simulink model "VVI"  (R2020a)
settings: Solver=FixedStepAuto  StartTime=0.0  StopTime=10.0  FixedStep=1e-3  RelTol=1e-3  EnableMultiTasking=on
undefined symbols (not defined in the file): D1, D10, D12, D13, D2, D3, D5, D7, D9, PTA1, PTA2, PTB9, PTC17, PTC3, PTC4, PTD0, PTD1, PTD3
libraries: frdmk64flib x11
settings Model: ExtModeTrigDuration=5  Creator=guga  LastModifiedBy=guga
settings OptimizationCC: EnhancedBackFolding=on  PassReuseOutputArgsAs=Individual arguments  ZeroExternalMemoryAtStartup=off  ZeroInternalMemoryAtStartup=off  MaxStackSize=64  OptimizeBlockOrder=speed  DifferentSizesBufferReuse=on  OptimizationCustomize=off  EfficientTunableParamExpr=on
settings DebuggingCC: ParameterTunabilityLossMsg=error
settings HardwareCC: ProdBitPerPointer=32  ProdBitPerSizeT=32  ProdBitPerPtrDiffT=32  ProdLargestAtomicInteger=Long  ProdLargestAtomicFloat=Double  ProdWordSize=32  ProdHWDeviceType=ARM Compatible->ARM Cortex
settings SFSimCC: MATLABDynamicMemAlloc=off
settings RTWCC: SystemTargetFile=ert.tlc  HardwareBoard=NXP FRDM-K64F  TemplateMakefile=ert_default_tmf  Toolchain=GNU Tools for ARM Embedded Processors
settings CodeAppCC: ForceParamTrailComments=on  IgnoreCustomStorageClasses=off  OperatorAnnotations=on  SimulinkDataObjDesc=on  SFDataObjDesc=on  InsertBlockDesc=on

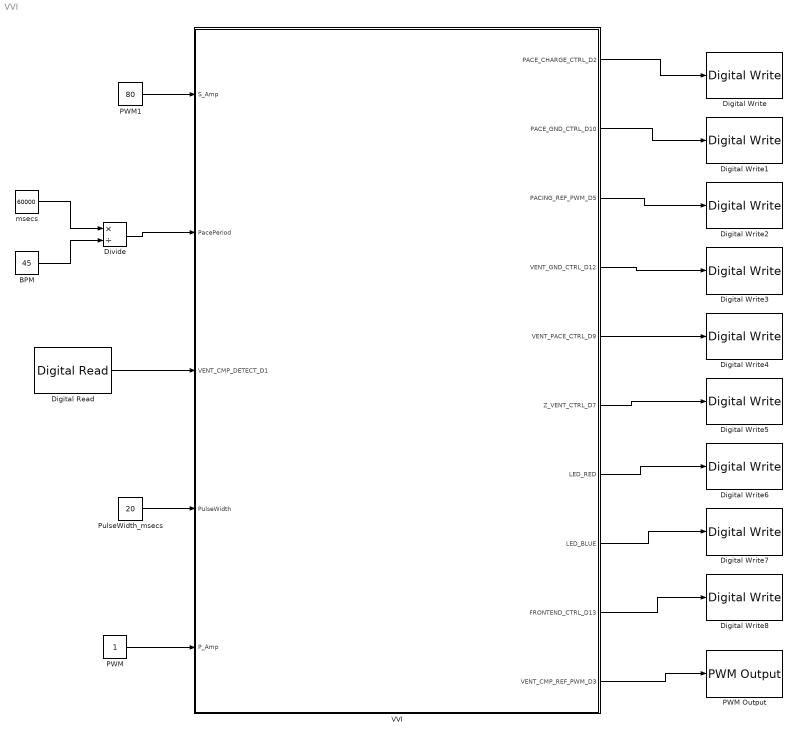
== system VVI ==
  BPM : Constant  Value=45
  Digital Read : frdmk64flib/Digital Read  Whichpin=PTC17 (D1)  SampleTime=-1
  Digital Write : frdmk64flib/Digital Write  Whichpin=PTB9 (D2)
  Digital Write1 : frdmk64flib/Digital Write  Whichpin=PTD0 (D10)
  Digital Write2 : frdmk64flib/Digital Write  Whichpin=PTA2 (D5)
  Digital Write3 : frdmk64flib/Digital Write  Whichpin=PTD3 (D12)
  Digital Write4 : frdmk64flib/Digital Write  Whichpin=PTC4 (D9)
  Digital Write5 : frdmk64flib/Digital Write  Whichpin=PTC3 (D7)
  Digital Write6 : frdmk64flib/Digital Write  Whichpin=RED_LED
  Digital Write7 : frdmk64flib/Digital Write  Whichpin=BLUE_LED
  Digital Write8 : frdmk64flib/Digital Write  Whichpin=PTD1 (D13)
  Divide : Product  Inputs=*/
  PWM : Constant
  PWM Output : frdmk64flib/PWM Output  Whichpin=PTA1 (D3)  InitialFrequency=2000  InitialDutyCycle=0
  PWM1 : Constant  Value=80
  PulseWidth_msecs : Constant  Value=20
  VVI : Stateflow chart  TreatAsAtomicUnit=on
  msecs : Constant  Value=60000
  wires:
  VVI/3(PACING_REF_PWM_D5) -> Digital Write2/1
  VVI/6(Z_VENT_CTRL_D7) -> Digital Write5/1
  VVI/7(LED_RED) -> Digital Write6/1
  VVI/1(PACE_CHARGE_CTRL_D2) -> Digital Write/1
  VVI/4(VENT_GND_CTRL_D12) -> Digital Write3/1
  VVI/2(PACE_GND_CTRL_D10) -> Digital Write1/1
  VVI/5(VENT_PACE_CTRL_D9) -> Digital Write4/1
  PWM/1 -> VVI/5(P_Amp)
  VVI/8(LED_BLUE) -> Digital Write7/1
  PWM1/1 -> VVI/1(S_Amp)
  Digital Read/1 -> VVI/3(VENT_CMP_DETECT_D1)
  VVI/9(FRONTEND_CTRL_D13) -> Digital Write8/1
  VVI/10(VENT_CMP_REF_PWM_D3) -> PWM Output/1
  Divide/1 -> VVI/2(PacePeriod)
  BPM/1 -> Divide/2
  msecs/1 -> Divide/1
  PulseWidth_msecs/1 -> VVI/4(PulseWidth)

== stateflow chart VVI/VVI ==
  state Pacing
    entry:
    PACING_REF_PWM_D5 = P_Amp;
    PACE_CHARGE_CTRL_D2 = 0;
    VENT_PACE_CTRL_D9 = 1;
    VENT_GND_CTRL_D12 = 0;
    PACE_GND_CTRL_D10 = 1;
    Z_VENT_CTRL_D7 = 0;
    LED_RED = 1;
    LED_BLUE = 0;
  state Charging_and_Sensing
    entry:
    PACING_REF_PWM_D5 = P_Amp;
    PACE_CHARGE_CTRL_D2 = 1;
    VENT_PACE_CTRL_D9 = 0;
    VENT_GND_CTRL_D12 = 1;
    PACE_GND_CTRL_D10 = 0;
    Z_VENT_CTRL_D7 = 0;
    LED_RED = 0;
    LED_BLUE = 1;
    FRONTEND_CTRL_D13 = 1;
    VENT_CMP_REF_PWM_D3 = S_Amp;
  (default) -> Charging_and_Sensing
  (junction 22) -> Charging_and_Sensing [order 1] : [VENT_CMP_DETECT_D1 == 1]
  Charging_and_Sensing -> (junction 22)
  (junction 22) -> Pacing [order 2] : after(PacePeriod-PulseWidth,msec)[VENT_CMP_DETECT_D1 == 0]
  Pacing -> Charging_and_Sensing : [after(PulseWidth,msec)]
  data: S_Amp input; PacePeriod input; VENT_CMP_DETECT_D1 input; PulseWidth input; P_Amp input; PACE_CHARGE_CTRL_D2 output; PACE_GND_CTRL_D10 output; PACING_REF_PWM_D5 output; VENT_GND_CTRL_D12 output; VENT_PACE_CTRL_D9 output; Z_VENT_CTRL_D7 output; LED_RED output; LED_BLUE output; FRONTEND_CTRL_D13 output; VENT_CMP_REF_PWM_D3 output
